simulink model "schema"  (R2013b)
settings: Solver=FixedStepDiscrete  StartTime=0.0  StopTime=0.0149  FixedStep=Te  RelTol=1e-3
values from neighbouring files (symbols this model uses):
  Te = 1e-4    (= 0.0001)    [script.m]
undefined symbols (not defined in the file or in its folder): den_pi, den_z, num_pi, num_z
settings Model: Creator=gemsdev  LastModifiedBy=gemsdev

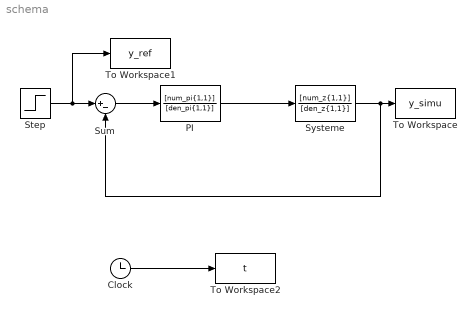
== system schema ==
  Clock : Clock
  PI : DiscreteTransferFcn  Numerator=[num_pi{1,1}]  Denominator=[den_pi{1,1}]  SampleTime=Te
  Step : Step  Time=0  SampleTime=0
  Sum : Sum  Inputs=|+-
  Systeme : DiscreteTransferFcn  Numerator=[num_z{1,1}]  Denominator=[den_z{1,1}]  SampleTime=Te
  To Workspace : ToWorkspace  VariableName=y_simu  SampleTime=-1
  To Workspace1 : ToWorkspace  VariableName=y_ref  SampleTime=-1
  To Workspace2 : ToWorkspace  VariableName=t  SampleTime=-1
  wires:
  PI/1 -> Systeme/1
  Step/1 -> To Workspace1/1, Sum/1
  Sum/1 -> PI/1
  Systeme/1 -> Sum/2, To Workspace/1
  Clock/1 -> To Workspace2/1
